simulink model "testLiniowosci"  (R2018a)
settings: Solver=VariableStepAuto  StartTime=0.0  StopTime=1000  RelTol=1e-3
values from neighbouring files (symbols this model uses):
  a = 8    [TAP_Projekt1.m]    (also in ZNExperiment.m; decoupling.m; matlab.mat; regInit.m)
  C = [1 0; 0 1]    [TAP_Projekt1.m]    (also in ZNExperiment.m = 0.4; decoupling.m = 0.4; matlab.mat = [1  0; 0  1]; regInit.m = 0.4)
  tau = 40    [TAP_Projekt1.m]    (also in ZNExperiment.m; decoupling.m; matlab.mat; regInit.m)
  tau_C = 100    [TAP_Projekt1.m]    (also in ZNExperiment.m; matlab.mat; regInit.m; tap_workspace.mat)
  TCp = 21    [TAP_Projekt1.m]    (also in ZNExperiment.m; decoupling.m; matlab.mat; regInit.m)
  TDp = 30    [TAP_Projekt1.m]    (also in ZNExperiment.m; decoupling.m; matlab.mat; regInit.m)
  THp = 64    [TAP_Projekt1.m]    (also in ZNExperiment.m; decoupling.m; matlab.mat; regInit.m)
settings Model: Creator=Barteux  LastModifiedBy=gajee
settings CodeAppCC: StateflowObjectComments=on

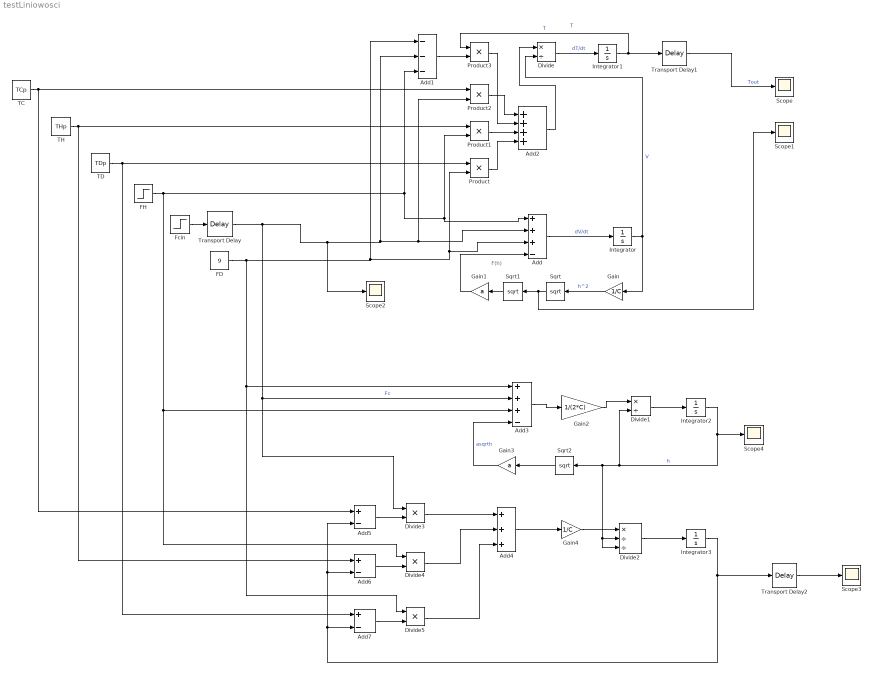
== system testLiniowosci ==
  note: T
  note: F(h)
  Add : Sum  Inputs=+++-
  Add1 : Sum  Inputs=---
  Add2 : Sum  Inputs=++++
  Add3 : Sum  Inputs=+++-
  Add4 : Sum  Inputs=+++
  Add5 : Sum  Inputs=+-
  Add6 : Sum  Inputs=+-
  Add7 : Sum  Inputs=+-
  Divide : Product  Inputs=*/
  Divide1 : Product  Inputs=*/
  Divide2 : Product  Inputs=*//
  Divide3 : Product  Inputs=**
  Divide4 : Product  Inputs=**
  Divide5 : Product  Inputs=**
  FD : Constant  Value=9
  FH : Step  Before=10  After=20  SampleTime=0
  Fcin : Step  Before=10  After=32  SampleTime=0
  Gain : Gain  Gain=1/C
  Gain1 : Gain  Gain=a
  Gain2 : Gain  Gain=1/(2*C)
  Gain3 : Gain  Gain=a
  Gain4 : Gain  Gain=1/C
  Integrator : Integrator  InitialCondition=1352
  Integrator1 : Integrator  InitialCondition=36.43
  Integrator2 : Integrator  InitialCondition=54
  Integrator3 : Integrator  InitialCondition=30
  Product{,1..3} (4 alike) : Product
  Scope{,1..4} (5 alike) : Scope
  Sqrt : Sqrt  SaturateOnIntegerOverflow=on
  Sqrt1 : Sqrt  SaturateOnIntegerOverflow=on
  Sqrt2 : Sqrt  SaturateOnIntegerOverflow=on
  TC : Constant  Value=TCp
  TD : Constant  Value=TDp
  TH : Constant  Value=THp
  Transport Delay : TransportDelay  DelayTime=tau_C
  Transport Delay1 : TransportDelay  DelayTime=tau
  Transport Delay2 : TransportDelay  DelayTime=tau
  wires:
  FH/1 -> Divide4/1, Add3/3, Add1/3, Add/1, Product1/2
  Fcin/1 -> Transport Delay/1
  FD/1 -> Divide5/1, Add3/1, Add1/1, Product/2, Add/3
  Add/1 -> Integrator/1  "dV/dt"
  Integrator/1 -> Gain/1, Divide/2  "V"
  Gain/1 -> Sqrt/1  "h^2"
  Sqrt/1 -> Scope1/1, Sqrt1/1
  Sqrt1/1 -> Gain1/1
  Gain1/1 -> Add/4
  TD/1 -> Add7/1, Product/1
  TH/1 -> Product1/1, Add6/1
  Add1/1 -> Product3/2
  Integrator1/1 -> Transport Delay1/1, Product3/1  "T"
  Divide/1 -> Integrator1/1  "dT/dt"
  Transport Delay/1 -> Divide3/1, Add3/2, Scope2/1, Add1/2, Product2/2, Add/2  "Fc"
  Transport Delay1/1 -> Scope/1  "Tout"
  Product2/1 -> Add2/1
  Product3/1 -> Add2/2
  Product1/1 -> Add2/3
  Product/1 -> Add2/4
  Add2/1 -> Divide/1
  Gain3/1 -> Add3/4  "asqrth"
  Add3/1 -> Gain2/1
  Gain2/1 -> Divide1/1
  Divide1/1 -> Integrator2/1
  Integrator2/1 -> Scope4/1, Divide2/3, Divide2/2, Sqrt2/1, Divide1/2  "h"
  Sqrt2/1 -> Gain3/1
  Gain4/1 -> Divide2/1
  Divide2/1 -> Integrator3/1
  Add4/1 -> Gain4/1
  Add5/1 -> Divide3/2
  Integrator3/1 -> Add7/2, Add6/2, Add5/2, Transport Delay2/1
  Divide3/1 -> Add4/1
  TC/1 -> Add5/1, Product2/1
  Divide4/1 -> Add4/2
  Divide5/1 -> Add4/3
  Add6/1 -> Divide4/2
  Add7/1 -> Divide5/2
  Transport Delay2/1 -> Scope3/1
